simulink model "IonistorDischargeTime"  (R2022b)
settings: Solver=VariableStepAuto  StartTime=0.0  StopTime=3.5*3600  FixedStep=60  RelTol=0.1  AbsTol=0.1
libraries: nesl_utility x3, fl_lib x3, ee_lib x2, simulink x1
settings Model: Creator=Vladimir  LastModifiedBy=Vladimir
settings SolverCC: ZeroCrossAlgorithm=Adaptive  AlgebraicLoopSolver=TrustRegion  MaxZcPerStep=1
settings OptimizationCC: BlockReduction=off  DefaultParameterBehavior=Inlined  BufferReuse=off
settings DebuggingCC: UnconnectedInputMsg=warning  UnconnectedOutputMsg=warning  UnconnectedLineMsg=warning  SymbolicDimsDataTypeCodeGenerationDiagnostic=none  SFMachineParentedDataDiag=warning
settings ModelReferenceCC: EnableRefExpFcnMdlSchedulingChecks=on
settings SFSimCC: CustomCodeUndefinedFunction=UseInterfaceOnly
settings RTWCC: DLArmComputeVersion=19.05
settings SimscapeCC: SimscapeLogType=all  SimscapeLogSimulationStatistics=on  SimscapeLogDataHistory=10000

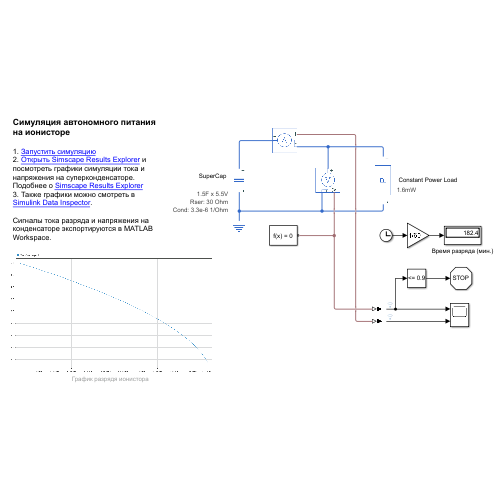
[thumbnail: Simulink's stored preview of the top-level diagram]
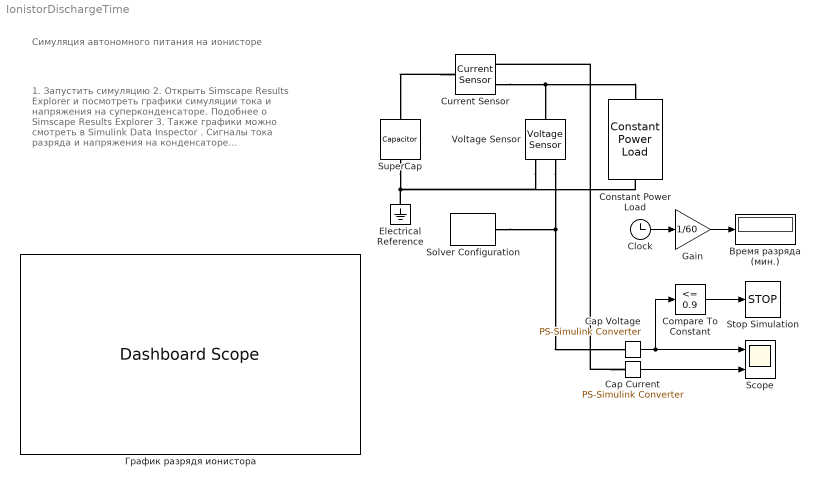
== system IonistorDischargeTime ==
  note: 1. Запустить симуляцию
      | 2. Открыть Simscape Results Explorer и посмотреть графики симуляции тока и напряжения на суперконденсаторе. Подобнее о Simscape Results Explorer
      | 3. Также графики можно смотреть в Simulink Data Inspector .
      |
      | Сигналы тока разряда и напряжения на конденсаторе экспортируются в MATLAB Workspace.
  note: Симуляция автономного питания на ионисторе
  Cap Current : nesl_utility/PS-Simulink Converter  PhysicalDomain=network_engine_domain  SubClassName=ps_output  LeftPortType=input  RightPortType=output  PseudoPeriodic=off  Frequencies=[]  VectorFormat=inherit  Unit=inherit  AffineConversion=off
  Cap Voltage : nesl_utility/PS-Simulink Converter  PhysicalDomain=network_engine_domain  SubClassName=ps_output  LeftPortType=input  RightPortType=output  PseudoPeriodic=off  Frequencies=[]  VectorFormat=inherit  Unit=inherit  AffineConversion=off
  Clock : Clock
  Compare To Constant : simulink/Logic and Bit Operations/Compare To Constant  relop=<=  const=0.9  OutDataTypeStr=boolean
  Constant Power Load : ee_lib/Passive/Constant Power Load  load_type=ee.enum.dc_ac.dc  consumed_power=1.6 mW  min_supply_voltage=0.8 V  G_reverse=1e-6 S  deltaV=1e-3 V  active_power=500 W  reactive_power=0 A*V  f0=60 Hz  Vrms_min=200 V  enable_fault=simscape.enum.onoff.off  fault_action=simscape.enum.assert.action.none  t_fault=1 s  open_conductance=1e-4 S
      settings: AttributesFormatString=%<consumed_power>%<consumed_power_unit>  InternalSimscapePortConfiguration="{\"Bottom\":[],\"Left\":[{\"id\":\"p\",\"label\":\"+\",\"type\":\"foundation.electrical.electrical\"}],\"Right\":[{\"id\":\"n\",\"label\":\"-\",\"type\":\"foundation.electrical.electrical\"}],\"Top\":[]}"
  Current Sensor : fl_lib/Electrical/Electrical Sensors/Current Sensor
  Electrical Reference : fl_lib/Electrical/Electrical Elements/Electrical Reference
  Gain : Gain  Gain=1/60
  Scope : Scope  NumInputPorts=2
  Solver Configuration : nesl_utility/Solver Configuration  PhysicalDomain=network_engine_domain  SubClassName=solver  LeftPortType=input  RightPortType=generic  Tones=[]  Harmonics=[]  SimulateNoise=off  Profile=off  UseLocalSampling=off  EnableSwitchedLinearOptims=on  FrequencyDomain=off  UseCCode=off  RelTol=0.001  AbsTol=1e-06  MinStep=1e-09  ToWorkspace=off  RevertToSquareIcSolve=off  NumHomotopyIterations=100  PhasorMode=off  PhasorModeNumHarmonics=1  ConsistencySolver=NEWTON_XTOL_AFTER_FTOL  IndexReductionMethod=DerivativeReplacement  DoDC=off  ResidualTolerance=1e-09  ConsistencyTolSource=GLOBAL  ConsistencyAbsTol=0.001  ConsistencyRelTol=0.001  ConsistencyTolFactor=0.1  UseLocalSolver=off  LocalSolverChoice=NE_BACKWARD_EULER_ADVANCER  ResolveIndetEquations=on  FunctionEvalNumThread=1  LocalSolverSampleTime=0.001  DoFixedCost=off  MaxNonlinIter=3  MaxModeIter=2  ComputeImpulses=off  ImpulseIterations=2  LinearAlgebra=auto  LinearAlgebraNumThread=0  EquationFormulation=NE_TIME_EF  DelaysMemoryBudget=1096  AutomaticFiltering=on  FilteringTimeConstant=0.1  PartitionStorageMethod=AS_NEEDED  PartitionMemoryBudget=1024  PartitionMethod=ROBUST
  Stop Simulation : Stop
  "SuperCap " : ee_lib/Passive/Capacitor  cap_option=0  c=1.5 F  Cvec=[1e-05, 1e-06] F  Vvec=[0, 10] V  CV_table_symmetry=1  f_vec=[1, 10] kHz  DFext_vec=[.8, 1.2]  enable_C_tol=0  C_tol=5  tol_distribution=1  nSigma=4  r=30 Ohm  g=3.3e-6 1/Ohm  averaging_period=0 s  enable_operating_limits=0  operating_limit_action=2  max_working_voltage_range=[-25, 25] V  power_rating=1 W  enable_faults=0  fault_action=1  Cscale_faulted=100  R_faulted=1e-3 Ohm  G_faulted=0 1/Ohm  tau_fault=1e-3 s  enable_temporal_fault=0  t_fault=1 s  enable_behavioral_fault=0  max_permissible_voltage_range=[-100, 100] V  t_fail_on_voltage=1 s  i_specify=off  i_priority=None  i=0 A  i_nominal_specify=on  i_nominal_unit=mA  i_nominal_value=350  v_specify=off  v_priority=High  v=2.7 V  v_nominal_specify=off  v_nominal_unit=V  v_nominal_value=1  vc_specify=on  vc_priority=High  vc=5 V  vc_nominal_specify=on  vc_nominal_unit=V  vc_nominal_value=5.5
      settings: LogSimulationData=on
      settings: AttributesFormatString=|
      | %<c>%<c_unit> x %<vc_nominal_value>%<vc_nominal_unit>
      | Rser: %<r> %<r_unit>
      | Cond: %<g> %<g_unit>
  Voltage Sensor : fl_lib/Electrical/Electrical Sensors/Voltage Sensor
  Время разряда (мин.) : Display
  График разрядя ионистора : DashboardScope  Ymin=0
  wires:
  Cap Voltage/1 -> Compare To Constant/1, Scope/1
  Compare To Constant/1 -> Stop Simulation/1
  Gain/1 -> Время разряда (мин.)/1
  Clock/1 -> Gain/1
  Cap Current/1 -> Scope/2
  connections:
  Electrical Reference/LConn1 -- Constant Power Load/RConn1 -- Voltage Sensor/RConn2 -- "SuperCap "/RConn1
  Current Sensor/RConn2 -- Voltage Sensor/LConn1 -- Constant Power Load/LConn1
  Voltage Sensor/RConn1 -- Cap Voltage/LConn1 -- Solver Configuration/RConn1
  Current Sensor/LConn1 -- "SuperCap "/LConn1
  Cap Current/LConn1 -- Current Sensor/RConn1
